simulink model "QPSK_Transmit"  (R2012b)
settings: Solver=FixedStepDiscrete  StartTime=0.0  StopTime=1000  RelTol=1e-3
libraries: simulink x21
settings Model: Creator=Carl  LastModifiedBy=Carl
settings DataIOCC: SignalLogging=off
settings OptimizationCC: BlockReduction=off  ConditionallyExecuteInputs=off  InlineParams=on
settings DebuggingCC: AlgebraicLoopMsg=error
settings HardwareCC: ProdHWDeviceType=ASIC/FPGA->ASIC/FPGA  ProdEqTarget=off

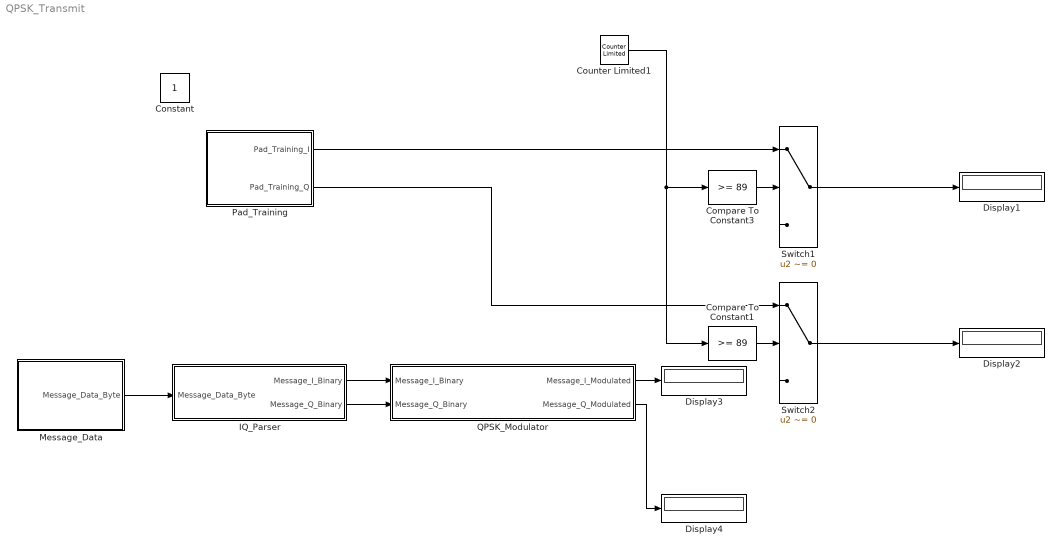
== system QPSK_Transmit ==
  Compare To Constant1 : simulink/Logic and Bit Operations/Compare To Constant  relop=>=  const=89  OutDataTypeStr=boolean  ZeroCross=off
  Compare To Constant3 : simulink/Logic and Bit Operations/Compare To Constant  relop=>=  const=89  OutDataTypeStr=boolean  ZeroCross=off
  Constant : Constant  OutDataTypeStr=boolean
  Counter Limited1 : simulink/Sources/Counter Limited  uplimit=1023  tsamp=-1
  Display{1..4} (4 alike) : Display
  IQ_Parser : Subsystem
  Message_Data : Subsystem
  Pad_Training : Subsystem
  QPSK_Modulator : Subsystem
  Switch1 : Switch  Criteria=u2 ~= 0
  Switch2 : Switch  Criteria=u2 ~= 0
  wires:
  Compare To Constant3/1 -> Switch1/2
  Counter Limited1/1 -> Compare To Constant1/1, Compare To Constant3/1
  Switch1/1 -> Display1/1
  Pad_Training/1(Pad_Training_I) -> Switch1/1
  Compare To Constant1/1 -> Switch2/2
  Switch2/1 -> Display2/1
  Pad_Training/2(Pad_Training_Q) -> Switch2/1
  Message_Data/1(Message_Data_Byte) -> IQ_Parser/1(Message_Data_Byte)
  IQ_Parser/1(Message_I_Binary) -> QPSK_Modulator/1(Message_I_Binary)
  IQ_Parser/2(Message_Q_Binary) -> QPSK_Modulator/2(Message_Q_Binary)
  QPSK_Modulator/1(Message_I_Modulated) -> Display3/1
  QPSK_Modulator/2(Message_Q_Modulated) -> Display4/1

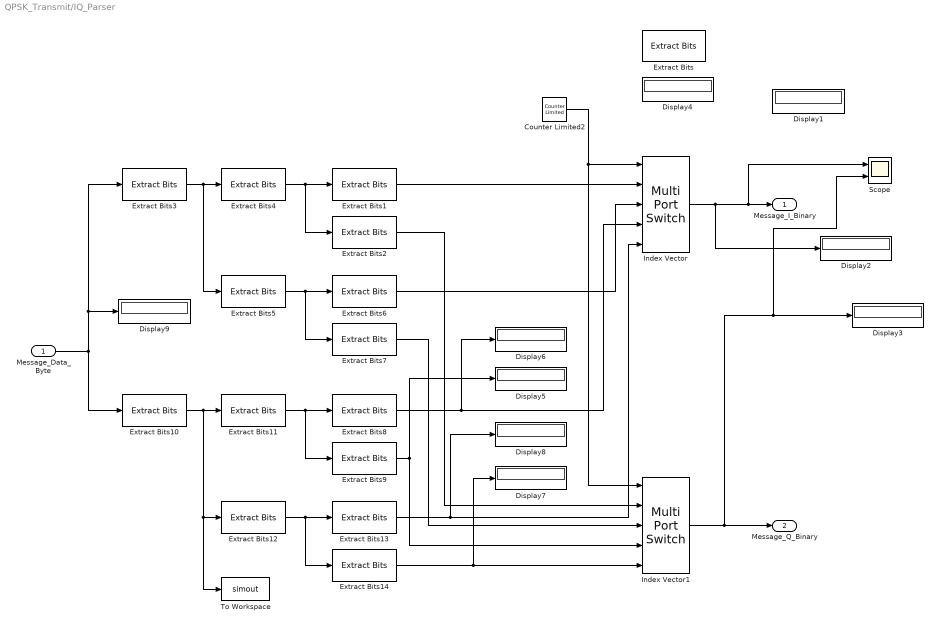
== system QPSK_Transmit/IQ_Parser ==
  Message_Data_Byte : Inport
  Counter Limited2 : simulink/Sources/Counter Limited  uplimit=3  tsamp=-1
  Display{1..9} (9 alike) : Display
  Extract Bits : simulink/Logic and Bit Operations/Extract Bits  bitsToExtract=Range starting with most significant bit  numBits=2  bitIdxRange=[15]  outScalingMode=Preserve fixed-point scaling
  Extract Bits{1,6,8,13} (4 alike) : simulink/Logic and Bit Operations/Extract Bits  bitsToExtract=Range starting with most significant bit  numBits=1  bitIdxRange=[15]  outScalingMode=Preserve fixed-point scaling
  Extract Bits10 : simulink/Logic and Bit Operations/Extract Bits  bitsToExtract=Lower half  numBits=2  bitIdxRange=[1 3 5 7]  outScalingMode=Preserve fixed-point scaling
  Extract Bits11 : simulink/Logic and Bit Operations/Extract Bits  bitsToExtract=Upper half  numBits=2  bitIdxRange=[0 2 4 6]  outScalingMode=Preserve fixed-point scaling
  Extract Bits12 : simulink/Logic and Bit Operations/Extract Bits  bitsToExtract=Lower half  numBits=2  bitIdxRange=[0 2 4 6]  outScalingMode=Preserve fixed-point scaling
  Extract Bits{2,7,9,14} (4 alike) : simulink/Logic and Bit Operations/Extract Bits  bitsToExtract=Range ending with least significant bit  numBits=1  bitIdxRange=[15]  outScalingMode=Preserve fixed-point scaling
  Extract Bits3 : simulink/Logic and Bit Operations/Extract Bits  bitsToExtract=Upper half  numBits=2  bitIdxRange=[0 2 4 6]  outScalingMode=Preserve fixed-point scaling
  Extract Bits4 : simulink/Logic and Bit Operations/Extract Bits  bitsToExtract=Upper half  numBits=2  bitIdxRange=[0 2 4 6]  outScalingMode=Preserve fixed-point scaling
  Extract Bits5 : simulink/Logic and Bit Operations/Extract Bits  bitsToExtract=Lower half  numBits=2  bitIdxRange=[0 2 4 6]  outScalingMode=Preserve fixed-point scaling
  Index Vector : MultiPortSwitch  DataPortOrder=Zero-based contiguous  Inputs=4  zeroidx=on
  Index Vector1 : MultiPortSwitch  DataPortOrder=Zero-based contiguous  Inputs=4  zeroidx=on
  Scope : Scope  NumInputPorts=2
      settings: YMin=-5~-5  YMax=5~5
  To Workspace : ToWorkspace  VariableName=simout  SampleTime=-1
  Message_I_Binary : Outport
  Message_Q_Binary : Outport  Port=2
  wires:
  Index Vector1/1 -> Scope/2, Display3/1, Message_Q_Binary/1
  Counter Limited2/1 -> Index Vector1/1, Index Vector/1
  Index Vector/1 -> Display2/1, Scope/1, Message_I_Binary/1
  Extract Bits3/1 -> Extract Bits5/1, Extract Bits4/1
  Extract Bits4/1 -> Extract Bits2/1, Extract Bits1/1
  Extract Bits5/1 -> Extract Bits6/1, Extract Bits7/1
  Extract Bits10/1 -> Extract Bits11/1, To Workspace/1, Extract Bits12/1
  Extract Bits11/1 -> Extract Bits8/1, Extract Bits9/1
  Extract Bits12/1 -> Extract Bits14/1, Extract Bits13/1
  Message_Data_Byte/1 -> Extract Bits10/1, Display9/1, Extract Bits3/1
  Extract Bits1/1 -> Index Vector/2
  Extract Bits2/1 -> Index Vector1/2
  Extract Bits6/1 -> Index Vector/3
  Extract Bits7/1 -> Index Vector1/3
  Extract Bits8/1 -> Display6/1, Index Vector/4
  Extract Bits9/1 -> Index Vector1/4, Display5/1
  Extract Bits13/1 -> Display8/1, Index Vector/5
  Extract Bits14/1 -> Display7/1, Index Vector1/5

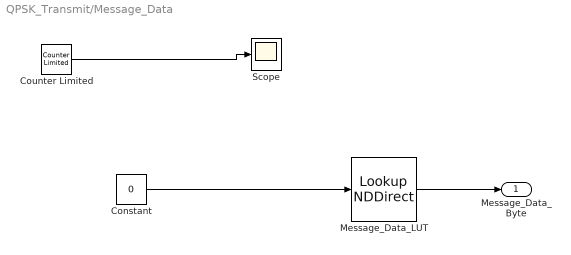
== system QPSK_Transmit/Message_Data ==
  Constant : Constant  Value=0
  Counter Limited : simulink/Sources/Counter Limited  uplimit=17  tsamp=-1
  Message_Data_LUT : LookupNDDirect  NumberOfTableDimensions=1  Table="[12        0        0        1        104        101        108        108        111        32        119        111        114        108        100        33        198        228]"  DiagnosticForOutOfRangeInput=Error  TableDataTypeStr=uint8
  Scope : Scope
  Message_Data_Byte : Outport
  wires:
  Message_Data_LUT/1 -> Message_Data_Byte/1
  Constant/1 -> Message_Data_LUT/1
  Counter Limited/1 -> Scope/1

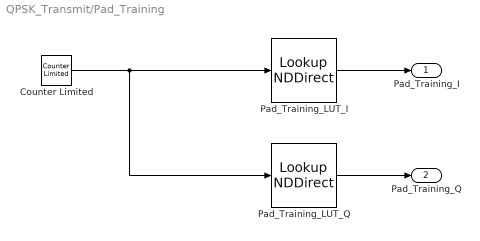
== system QPSK_Transmit/Pad_Training ==
  Counter Limited : simulink/Sources/Counter Limited  uplimit=89  tsamp=-1
  Pad_Training_LUT_I : LookupNDDirect  NumberOfTableDimensions=1  Table=[1,-1,1,-1,1,-1,1,-1,1,-1,1,-1,1,-1,1,-1,1,-1,1,-1,1,-1,1,-1,1,1,1,-1,-1,1,1,-1,-1,1,-1,-1,-1,-1,1,-1,1,1,-1,-1,1,1,1,-1,1,1,1,-1,1,-1,1,1,1,-1,1,1,1,1,-1,1,1,-1,-1,-1,-1,1,1,1,-1,-1,-1,1,1,1,1,-1,1,1,1,1,1,-1,-1,-1,1,1]  DiagnosticForOutOfRangeInput=Error  TableDataTypeStr=int8
  Pad_Training_LUT_Q : LookupNDDirect  NumberOfTableDimensions=1  Table=[1,-1,1,-1,1,-1,1,-1,1,-1,1,-1,1,-1,1,-1,1,-1,1,-1,1,-1,1,-1,1,1,-1,1,1,1,-1,-1,-1,-1,1,1,-1,1,1,-1,-1,-1,1,-1,-1,1,1,1,-1,-1,1,1,1,-1,-1,-1,-1,-1,-1,1,1,-1,1,-1,1,1,-1,-1,1,-1,-1,1,1,-1,-1,-1,-1,-1,1,1,1,1,-1,-1,-1,-1,1,-1,1,-1]  DiagnosticForOutOfRangeInput=Error  TableDataTypeStr=int8
  Pad_Training_I : Outport
  Pad_Training_Q : Outport  Port=2
  wires:
  Pad_Training_LUT_I/1 -> Pad_Training_I/1
  Counter Limited/1 -> Pad_Training_LUT_I/1, Pad_Training_LUT_Q/1
  Pad_Training_LUT_Q/1 -> Pad_Training_Q/1

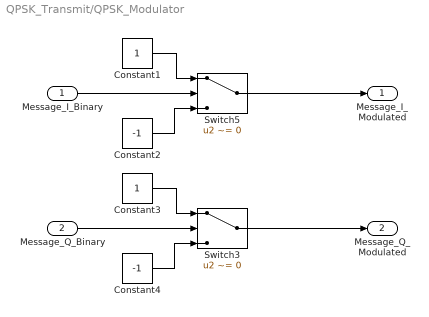
== system QPSK_Transmit/QPSK_Modulator ==
  Message_I_Binary : Inport
  Message_Q_Binary : Inport  Port=2
  Constant1 : Constant  OutDataTypeStr=boolean
  Constant2 : Constant  Value=-1  OutDataTypeStr=boolean
  Constant3 : Constant  OutDataTypeStr=boolean
  Constant4 : Constant  Value=-1  OutDataTypeStr=boolean
  Switch3 : Switch  Criteria=u2 ~= 0  RndMeth=Round
  Switch5 : Switch  Criteria=u2 ~= 0  RndMeth=Round
  Message_I_Modulated : Outport
  Message_Q_Modulated : Outport  Port=2
  wires:
  Switch3/1 -> Message_Q_Modulated/1
  Constant4/1 -> Switch3/3
  Constant2/1 -> Switch5/3
  Constant1/1 -> Switch5/1
  Message_Q_Binary/1 -> Switch3/2
  Constant3/1 -> Switch3/1
  Switch5/1 -> Message_I_Modulated/1
  Message_I_Binary/1 -> Switch5/2
